simulink model "hhs_model_vs8_2018b"  (R2018b)
settings: Solver=ode23  StartTime=0.0  StopTime=365*24*3600  MaxStep=3600  RelTol=1e-3
undefined symbols (not defined in the file or in its folder): A, B, C, D
libraries: simulink_need_slupdate x1
settings Model: ExtModeTrigMode=oneshot  ExtModeArmWhenConnect=off  Creator=Arie Taal  LastModifiedBy=Uitleen
settings DataIOCC: LimitDataPoints=on  SaveFormat=Array
settings OptimizationCC: BlockReduction=off  BooleanDataType=off  LifeSpan=inf
settings DebuggingCC: SaveWithParameterizedLinksMsg=none  UnderspecifiedInitializationDetection=Classic  MergeDetectMultiDrivingBlocksExec=none  SignalResolutionControl=TryResolveAllWithWarning  SFUnexpectedBacktrackingDiag=warning  SFNoUnconditionalDefaultTransitionDiag=warning  SFExecutionAtInitializationDiag=none
settings HardwareCC: ProdBitPerPointer=32  ProdBitPerSizeT=32  ProdBitPerPtrDiffT=32  ProdLargestAtomicFloat=None  ProdIntDivRoundTo=Undefined  ProdEndianess=Unspecified  ProdWordSize=32  ProdHWDeviceType=32-bit Generic  TargetUnknown=on
settings ModelReferenceCC: PropagateSignalLabelsOutOfModel=off
settings SFSimCC: SimUseLocalCustomCode=off
settings RTWCC: RTWUseLocalCustomCode=off
settings CodeAppCC: StateflowObjectComments=on
settings GRTTargetCC: TargetLangStandard=C89/C90 (ANSI)  GeneratePreprocessorConditionals=Disable all
settings ConfigComp: CovMetricSettings=dw  CovHtmlReporting=on  CovSaveCumulativeToWorkspaceVar=on  CovSaveSingleToWorkspaceVar=on  CovExternalEMLEnable=off  CovSFcnEnable=off

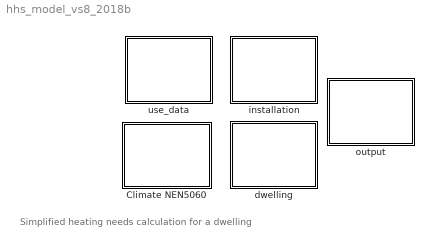
== system hhs_model_vs8_2018b ==
  note: Simplified heating needs calculation for a dwelling
  Climate NEN5060 : Subsystem  mask(Climate){ntype=Typical meteorological year (to be used for energy calculations)}
      mask help:
      | NEN5060:2008
      | assumption: no solar radiation by ground reflection.
      mask init:
      | if ntype==1
      | load NEN5060_A2 
      | elseif ntype==2
      | load NEN5060_B2_1
      | elseif ntype==3
      | load NEN5060_B2_2
      | elseif ntype==4
      | load NEN5060_B2_3
      | end
      mask Help:
      | Data from NEN5060:2008 is loaded.
      | NEN5060 consists of 2 kind of files:
      | A - for calculation of the energy demand
      | B - for calculation of indoor temperature
      | 
      | Furthermore, in case of calculation of indoor temperature the files are
      | divided in probabilities of 1, 2 and 5 %.
      mask TypeOptions ntype: Typical meteorological year (to be used for energy calculations) | 1 % deviation | 2 % deviation | 5 % deviation
      mask DialogControl DescGroupVar Prompt: Climate NEN5060:2018
      mask DialogControl Control3 Prompt: Climate data selection
      mask Display: disp('Climate data')
  dwelling : Subsystem  mask(dwelling){A_facade=160.2, Rc_facade=1.3, glass=[9.5 9.5 0 0 0 0 0 0], Uglass=2.9, g_value=0.7, CF=0.8, n=0.55, V_dwelling=275.6, N_facade=Middle weight, A_internal_mass=106+64, N_internal_mass=Middle weight}
      mask prompts: A_facade "Envelope surface (facade + roof + ground) [m2]"; Rc_facade "Envelope thermal resitance, R-value [m2/KW]"; glass "Windows surface [N,S,E,W,SE,SW,NE,NW] [m2]"; Uglass "Window thermal transmittance, U-value [W/m2K]"; g_value "Window solar transmitance, g-value"; n "Ventilation, air changes per hour [#/h]"; V_dwelling "Internal volume [m3]"; N_facade "Facade construction"; A_internal_mass "Floor and internal walls surface [m2]"; N_internal_mass "Floor and internal walls construction"
      mask init:
      | init_dwelling
      mask TypeOptions N_facade: Light weight | Middle weight | Heavy weight
      mask TypeOptions N_internal_mass: Light weight | Middle weight | Heavy weight
      mask DialogControl Control2 Prompt: Dwelling characteristics
      mask Display: disp('Dwelling')
  installation : Subsystem  mask(installation){Pheat=12000, P=10000, I=0, D=0}
      mask prompts: Pheat "Nominal heating capacity [W]"; P "Proportional"; I "Integral"; D "Derivative"
      mask DialogControl Container7 Prompt: Installatie
      mask DialogControl Container10 Prompt: PID controller
      mask Display: disp('Installation')
  output : Subsystem  mask(output){}
      mask Display: disp('Output')
  use_data : Subsystem  mask(use_data){Tday=20, DeltaT=5, Qday=150, DeltaQ=100, t1=8, t2=23}
      mask prompts: Tday "Day setpoint temperature [ºC]"; DeltaT "Temperature difference between day and night setpoint  [ºC]"; Qday "Day internal heat gains [W]"; DeltaQ "Internal heat gains difference between day and night"; t1 "Presence from [hour]"; t2 "Presence until [hour]"
      mask DialogControl DescTextVar Prompt: USE DATA
      mask DialogControl Control2 Prompt: - the schedule is for all days the same
      mask DialogControl Control3 Prompt: - day and night setpoint temperature and Q internal  related to presence schedule
      mask Display: disp('Dwelling use data')

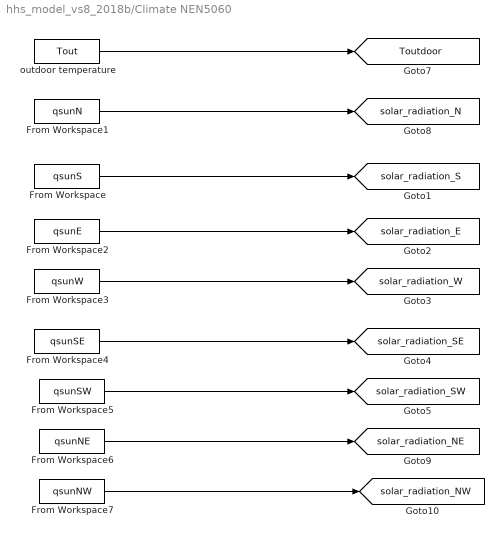
== system hhs_model_vs8_2018b/Climate NEN5060 ==
  From Workspace : FromWorkspace  VariableName=qsunS  SampleTime=0
  From Workspace1 : FromWorkspace  VariableName=qsunN  SampleTime=0
  From Workspace2 : FromWorkspace  VariableName=qsunE  SampleTime=0
  From Workspace3 : FromWorkspace  VariableName=qsunW  SampleTime=0
  From Workspace4 : FromWorkspace  VariableName=qsunSE  SampleTime=0
  From Workspace5 : FromWorkspace  VariableName=qsunSW  SampleTime=0
  From Workspace6 : FromWorkspace  VariableName=qsunNE  SampleTime=0
  From Workspace7 : FromWorkspace  VariableName=qsunNW  SampleTime=0
  outdoor temperature : FromWorkspace  VariableName=Tout  SampleTime=0
  tag scope: Toutdoor=global, solar_radiation_E=global, solar_radiation_N=global, solar_radiation_NE=global, solar_radiation_NW=global, solar_radiation_S=global, solar_radiation_SE=global, solar_radiation_SW=global, solar_radiation_W=global
  wires:
  outdoor temperature/1 -> [Toutdoor]
  From Workspace1/1 -> [solar_radiation_N]
  From Workspace/1 -> [solar_radiation_S]
  From Workspace2/1 -> [solar_radiation_E]
  From Workspace3/1 -> [solar_radiation_W]
  From Workspace4/1 -> [solar_radiation_SE]
  From Workspace5/1 -> [solar_radiation_SW]
  From Workspace6/1 -> [solar_radiation_NE]
  From Workspace7/1 -> [solar_radiation_NW]

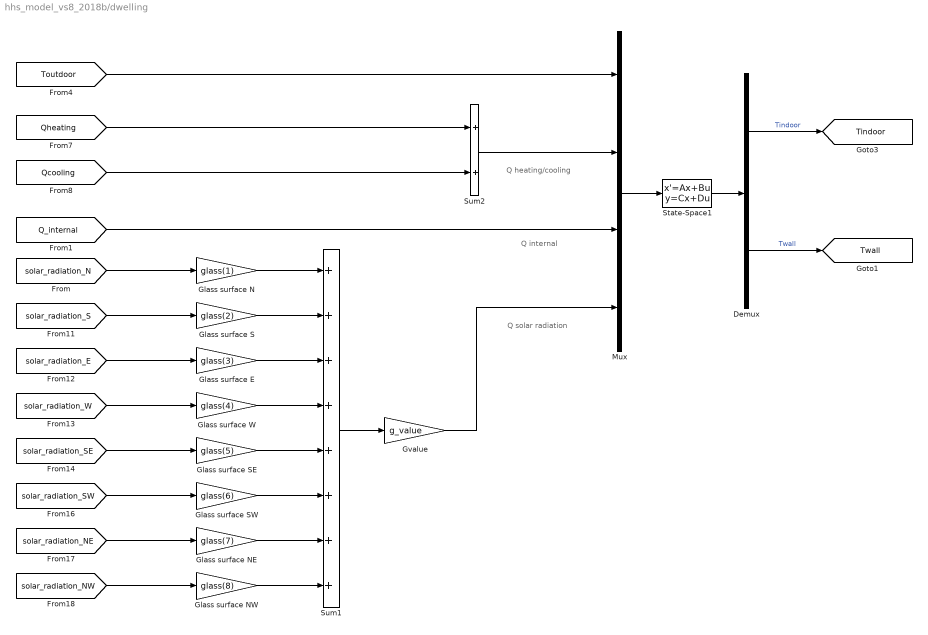
== system hhs_model_vs8_2018b/dwelling ==
  note: Q heating/cooling
  note: Q internal
  note: Q solar radiation
  Demux : Demux  Outputs=2
  Glass surface E : Gain  Gain=glass(3)  SaturateOnIntegerOverflow=on  OutDataTypeStr=Inherit: Same as input  ParamDataTypeStr=Inherit: Same as input
  Glass surface N : Gain  Gain=glass(1)  SaturateOnIntegerOverflow=on  OutDataTypeStr=Inherit: Same as input  ParamDataTypeStr=Inherit: Same as input
  Glass surface NE : Gain  Gain=glass(7)  SaturateOnIntegerOverflow=on  OutDataTypeStr=Inherit: Same as input  ParamDataTypeStr=Inherit: Same as input
  Glass surface NW : Gain  Gain=glass(8)  SaturateOnIntegerOverflow=on  OutDataTypeStr=Inherit: Same as input  ParamDataTypeStr=Inherit: Same as input
  Glass surface S : Gain  Gain=glass(2)  SaturateOnIntegerOverflow=on  OutDataTypeStr=Inherit: Same as input  ParamDataTypeStr=Inherit: Same as input
  Glass surface SE : Gain  Gain=glass(5)  SaturateOnIntegerOverflow=on  OutDataTypeStr=Inherit: Same as input  ParamDataTypeStr=Inherit: Same as input
  Glass surface SW : Gain  Gain=glass(6)  SaturateOnIntegerOverflow=on  OutDataTypeStr=Inherit: Same as input  ParamDataTypeStr=Inherit: Same as input
  Glass surface W : Gain  Gain=glass(4)  SaturateOnIntegerOverflow=on  OutDataTypeStr=Inherit: Same as input  ParamDataTypeStr=Inherit: Same as input
  Gvalue : Gain  Gain=g_value  SaturateOnIntegerOverflow=on  OutDataTypeStr=Inherit: Same as input  ParamDataTypeStr=Inherit: Same as input
  Mux : Mux
  State-Space1 : StateSpace  A=A  B=B  C=C  D=D  InitialCondition=0
  Sum1 : Sum  Inputs=++++++++  SaturateOnIntegerOverflow=on  InputSameDT=on  OutDataTypeStr=Inherit: Same as first input
  Sum2 : Sum  SaturateOnIntegerOverflow=on  InputSameDT=on  OutDataTypeStr=Inherit: Same as first input
  tag scope: Tindoor=global, Twall=global
  wires:
  Mux/1 -> State-Space1/1
  State-Space1/1 -> Demux/1
  Sum2/1 -> Mux/2
  Demux/1 -> [Tindoor]  "Tindoor"
  [Qheating] -> Sum2/1
  [Qcooling] -> Sum2/2
  [solar_radiation_S] -> Glass surface S/1
  [solar_radiation_E] -> Glass surface E/1
  [solar_radiation_W] -> Glass surface W/1
  [solar_radiation_SE] -> Glass surface SE/1
  [solar_radiation_SW] -> Glass surface SW/1
  [solar_radiation_NE] -> Glass surface NE/1
  [solar_radiation_NW] -> Glass surface NW/1
  Glass surface N/1 -> Sum1/1
  Glass surface S/1 -> Sum1/2
  Glass surface E/1 -> Sum1/3
  Glass surface W/1 -> Sum1/4
  Glass surface SE/1 -> Sum1/5
  Glass surface SW/1 -> Sum1/6
  Glass surface NE/1 -> Sum1/7
  Glass surface NW/1 -> Sum1/8
  Sum1/1 -> Gvalue/1
  Gvalue/1 -> Mux/4
  [Q_internal] -> Mux/3
  [Toutdoor] -> Mux/1
  [solar_radiation_N] -> Glass surface N/1
  Demux/2 -> [Twall]  "Twall"

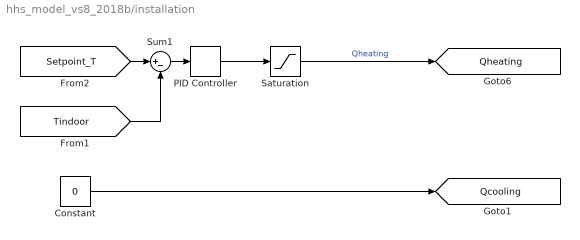
== system hhs_model_vs8_2018b/installation ==
  Constant : Constant  Value=0
  PID Controller : simulink_need_slupdate/PID Controller  P=P  I=I  D=D
      settings: SourceProductName=Simulink
  Saturation : Saturate  UpperLimit=Pheat  LowerLimit=0
  Sum1 : Sum  Inputs=|+-  SaturateOnIntegerOverflow=on  InputSameDT=on  OutDataTypeStr=Inherit: Same as first input
  tag scope: Qcooling=global, Qheating=global
  wires:
  [Tindoor] -> Sum1/2
  [Setpoint_T] -> Sum1/1
  Sum1/1 -> PID Controller/1
  PID Controller/1 -> Saturation/1
  Constant/1 -> [Qcooling]
  Saturation/1 -> [Qheating]  "Qheating"

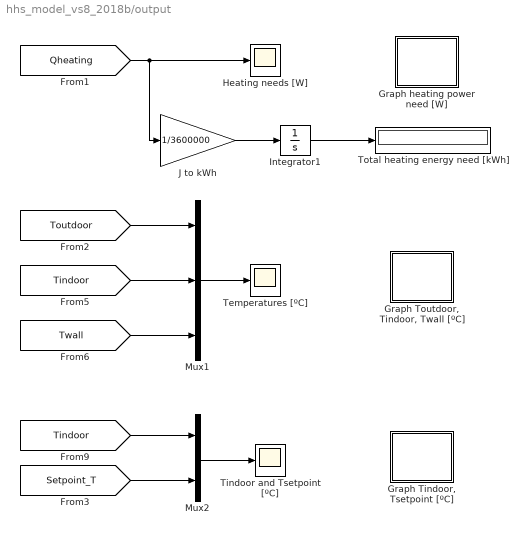
== system hhs_model_vs8_2018b/output ==
  "Graph Tindoor, Tsetpoint [ºC]" : Subsystem
      settings: OpenFcn=graph_tin_tsetpoint
  "Graph Toutdoor, Tindoor, Twall [ºC]" : Subsystem
      settings: OpenFcn=graph_tout_tin_twall
  Graph heating power need [W] : Subsystem
      settings: OpenFcn=graph_heating_needs
  Heating needs [W] : Scope
  Integrator1 : Integrator
  J to kWh : Gain  Gain=1/3600000  SaturateOnIntegerOverflow=on  OutDataTypeStr=Inherit: Same as input  ParamDataTypeStr=Inherit: Same as input
  Mux1 : Mux  Inputs=3
  Mux2 : Mux  Inputs=2
  Temperatures [ºC] : Scope
  Tindoor and Tsetpoint [ºC] : Scope
  Total heating energy need [kWh] : Display
  wires:
  Mux1/1 -> Temperatures [ºC]/1
  [Setpoint_T] -> Mux2/2
  [Tindoor] -> Mux1/2
  Mux2/1 -> Tindoor and Tsetpoint [ºC]/1
  [Tindoor] -> Mux2/1
  [Twall] -> Mux1/3
  [Toutdoor] -> Mux1/1
  Integrator1/1 -> Total heating energy need [kWh]/1
  [Qheating] -> J to kWh/1, Heating needs [W]/1
  J to kWh/1 -> Integrator1/1

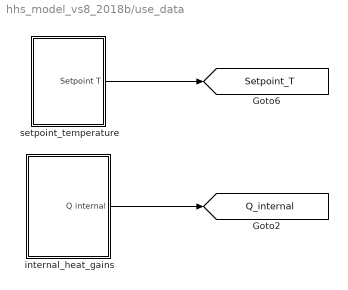
== system hhs_model_vs8_2018b/use_data ==
  internal_heat_gains : Subsystem  mask(internal_heat_gains){NightQ=Qday-DeltaQ, DeltaQ=DeltaQ}
      mask prompts: NightQ "Night Q internal  [W]"; DeltaQ "Day Delta Q internal [W]"
      mask Display: disp('Internal heat\n gains')
  setpoint_temperature : Subsystem  mask(setpoint_temperature){NightT=Tday-DeltaT, DeltaT=DeltaT}
      mask prompts: NightT "Night setpoint temperature [oC]"; DeltaT "Delta T, day-night setpoint temperature difference  [oC]"
      mask Display: disp('Setpoint\n temperature')
  tag scope: Q_internal=global, Setpoint_T=global
  wires:
  setpoint_temperature/1(Setpoint T) -> [Setpoint_T]
  internal_heat_gains/1(Q internal) -> [Q_internal]

== system hhs_model_vs8_2018b/output/Graph Tindoor, Tsetpoint [ºC] ==

== system hhs_model_vs8_2018b/output/Graph Toutdoor, Tindoor, Twall [ºC] ==

== system hhs_model_vs8_2018b/output/Graph heating power need [W] ==

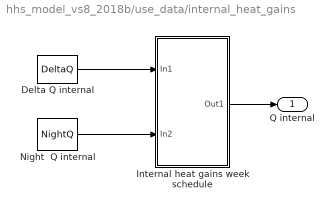
== system hhs_model_vs8_2018b/use_data/internal_heat_gains ==
  Delta Q internal : Constant  Value=DeltaQ
  Internal heat gains week schedule : Subsystem
  Night  Q internal : Constant  Value=NightQ
  Q internal : Outport
  wires:
  Internal heat gains week schedule/1(Out1) -> Q internal/1
  Night  Q internal/1 -> Internal heat gains week schedule/2(In2)
  Delta Q internal/1 -> Internal heat gains week schedule/1(In1)

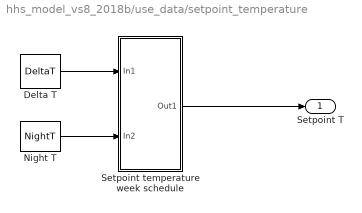
== system hhs_model_vs8_2018b/use_data/setpoint_temperature ==
  Delta T : Constant  Value=DeltaT
  Night T : Constant  Value=NightT
  Setpoint temperature week schedule : Subsystem
  Setpoint T : Outport
  wires:
  Delta T/1 -> Setpoint temperature week schedule/1(In1)
  Night T/1 -> Setpoint temperature week schedule/2(In2)
  Setpoint temperature week schedule/1(Out1) -> Setpoint T/1

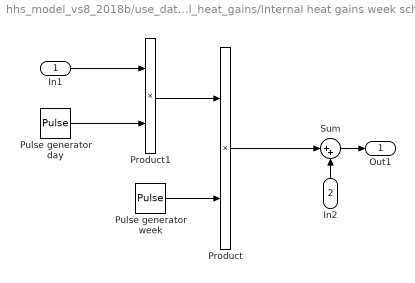
== system hhs_model_vs8_2018b/use_data/internal_heat_gains/Internal heat gains week schedule ==
  In1 : Inport
  In2 : Inport  Port=2
  Product : Product  SaturateOnIntegerOverflow=on  RndMeth=Zero  InputSameDT=on  OutDataTypeStr=Inherit: Same as first input
  Product1 : Product  SaturateOnIntegerOverflow=on  RndMeth=Zero  InputSameDT=on  OutDataTypeStr=Inherit: Same as first input
  Pulse generator day : DiscretePulseGenerator  PulseType=Time based  Period=24*3600  PulseWidth=(t2-t1)/24*100  PhaseDelay=t1*3600
  Pulse generator week : DiscretePulseGenerator  PulseType=Time based  Period=7*24*3600  PulseWidth=99.99
  Sum : Sum  Inputs=|++  SaturateOnIntegerOverflow=on  InputSameDT=on  OutDataTypeStr=Inherit: Same as first input
  Out1 : Outport
  wires:
  In2/1 -> Sum/2
  Sum/1 -> Out1/1
  In1/1 -> Product1/1
  Product1/1 -> Product/1
  Pulse generator day/1 -> Product1/2
  Pulse generator week/1 -> Product/2
  Product/1 -> Sum/1

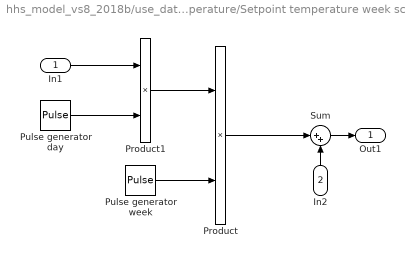
== system hhs_model_vs8_2018b/use_data/setpoint_temperature/Setpoint temperature week schedule ==
  In1 : Inport
  In2 : Inport  Port=2
  Product : Product  SaturateOnIntegerOverflow=on  RndMeth=Zero  InputSameDT=on  OutDataTypeStr=Inherit: Same as first input
  Product1 : Product  SaturateOnIntegerOverflow=on  RndMeth=Zero  InputSameDT=on  OutDataTypeStr=Inherit: Same as first input
  Pulse generator day : DiscretePulseGenerator  PulseType=Time based  Period=24*3600  PulseWidth=(t2-t1)/24*100  PhaseDelay=t1*3600
  Pulse generator week : DiscretePulseGenerator  PulseType=Time based  Period=7*24*3600  PulseWidth=99.99
  Sum : Sum  Inputs=|++  SaturateOnIntegerOverflow=on  InputSameDT=on  OutDataTypeStr=Inherit: Same as first input
  Out1 : Outport
  wires:
  Product/1 -> Sum/1
  Pulse generator week/1 -> Product/2
  Pulse generator day/1 -> Product1/2
  Product1/1 -> Product/1
  In1/1 -> Product1/1
  Sum/1 -> Out1/1
  In2/1 -> Sum/2
